simulink model "PANCd"  (R2020a)
settings: Solver=ode3  StartTime=0.0  StopTime=10.0  FixedStep=0.1  RelTol=1e-3  EnableMultiTasking=on
settings Model: Creator=CARVALHO  LastModifiedBy=Arnaldo
settings DataIOCC: LimitDataPoints=on  SaveFormat=Array  ReturnWorkspaceOutputs=off
settings OptimizationCC: LifeSpan=inf
settings DebuggingCC: SFUnexpectedBacktrackingDiag=warning  SFNoUnconditionalDefaultTransitionDiag=warning  SFExecutionAtInitializationDiag=none  ArithmeticOperatorsInVariantConditions=warning
settings HardwareCC: ProdBitPerPointer=32  ProdBitPerSizeT=32  ProdBitPerPtrDiffT=32  ProdLargestAtomicFloat=None  ProdIntDivRoundTo=Undefined  ProdEndianess=Unspecified  ProdWordSize=32  ProdHWDeviceType=32-bit Generic
settings ModelReferenceCC: PropagateSignalLabelsOutOfModel=off
settings SFSimCC: SimUseLocalCustomCode=off  CustomCodeUndefinedFunction=UseInterfaceOnly
settings RTWCC: RTWUseLocalCustomCode=off
settings CodeAppCC: StateflowObjectComments=on
settings GRTTargetCC: TargetLangStandard=C89/C90 (ANSI)
settings ConfigComp: CovMetricSettings=dw  CovHtmlReporting=on  CovSaveCumulativeToWorkspaceVar=on  CovSaveSingleToWorkspaceVar=on  CovExternalEMLEnable=off

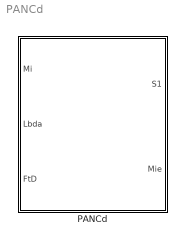
== system PANCd ==
  PANCd : Subsystem  Tag=NAP  Description=Célula de Aprendizagem NAP

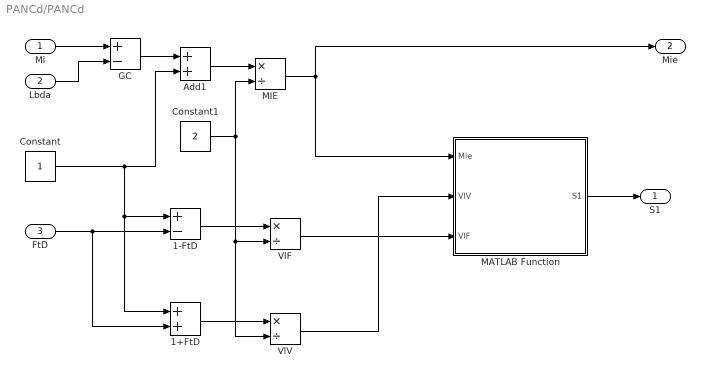
== system PANCd/PANCd ==
  Mi : Inport
  Lbda : Inport  Port=2
  FtD : Inport  Port=3
  1+FtD : Sum
  1-FtD : Sum  Inputs=+-
  Add1 : Sum
  Constant : Constant
  Constant1 : Constant  Value=2
  GC : Sum  Inputs=+-
  MATLAB Function : MATLAB Function  TreatAsAtomicUnit=on
  MIE : Product  Inputs=*/
  VlF : Product  Inputs=*/
  VlV : Product  Inputs=*/
  S1 : Outport
  Mie : Outport  Port=2
  wires:
  Mi/1 -> GC/1
  GC/1 -> Add1/1
  Add1/1 -> MIE/1
  Constant1/1 -> VlV/2, VlF/2, MIE/2
  Constant/1 -> 1-FtD/1, 1+FtD/1, Add1/2
  FtD/1 -> 1+FtD/2, 1-FtD/2
  1-FtD/1 -> VlF/1
  1+FtD/1 -> VlV/1
  MIE/1 -> MATLAB Function/1(Mie), Mie/1
  Lbda/1 -> GC/2
  VlV/1 -> MATLAB Function/2(VlV)
  MATLAB Function/1(S1) -> S1/1
  VlF/1 -> MATLAB Function/3(VlF)

== matlab function PANCd/MATLAB Function ==
  data: Mie input; S1 output; VlV input; VlF input
function S1 = fcn(Mie, VlV, VlF)
%#codegen
if Mie>=VlV
    S1=1;
else if Mie<=VlF
        S1=0;
    else 
        S1=0.5;
    end
end
